simulink model "LQR_control_Xmotion"  (R2025b)
settings: Solver=VariableStepAuto  StartTime=0.0  StopTime=10.0  RelTol=1e-3
values from neighbouring files (symbols this model uses):
  A_Mat = [ 0     1    0     0   0   0 ... (first row only)    [LQR_code_XYmotion.m]    (also in LQR_code_Xmotion.m = [ 0     1    0     0; LQR_control_AND_Plant2026.m = [ 0     1    0     0)
  B_Mat = [ 0    0 ... (first row only)    [LQR_code_XYmotion.m]    (also in LQR_code_Xmotion.m = [ 0; LQR_control_AND_Plant2026.m = [ 0)
  C_Mat = [ 1  0    0   0   0  0 ... (first row only)    [LQR_code_XYmotion.m]    (also in LQR_code_Xmotion.m = [ 1  0    0   0; LQR_control_AND_Plant2026.m = [ 1  0    0   0)
  K = lqr(A_Mat, B_Mat, Q, R)    [LQR_code_XYmotion.m]    (also in LQR_code_Xmotion.m; LQR_control_AND_Plant2026.m)
settings Model: Creator=Mahmoud Essam  LastModifiedBy=Mahmoud Essam

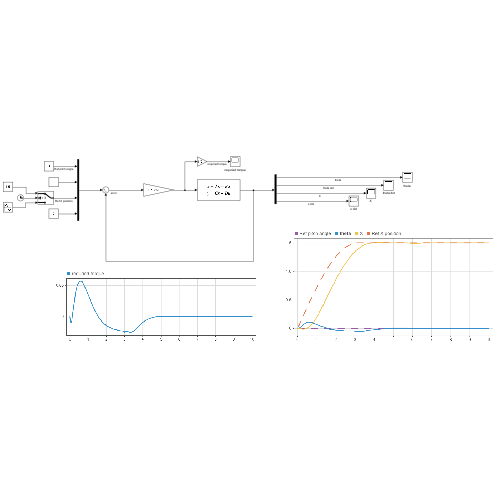
[thumbnail: Simulink's stored preview of the top-level diagram]
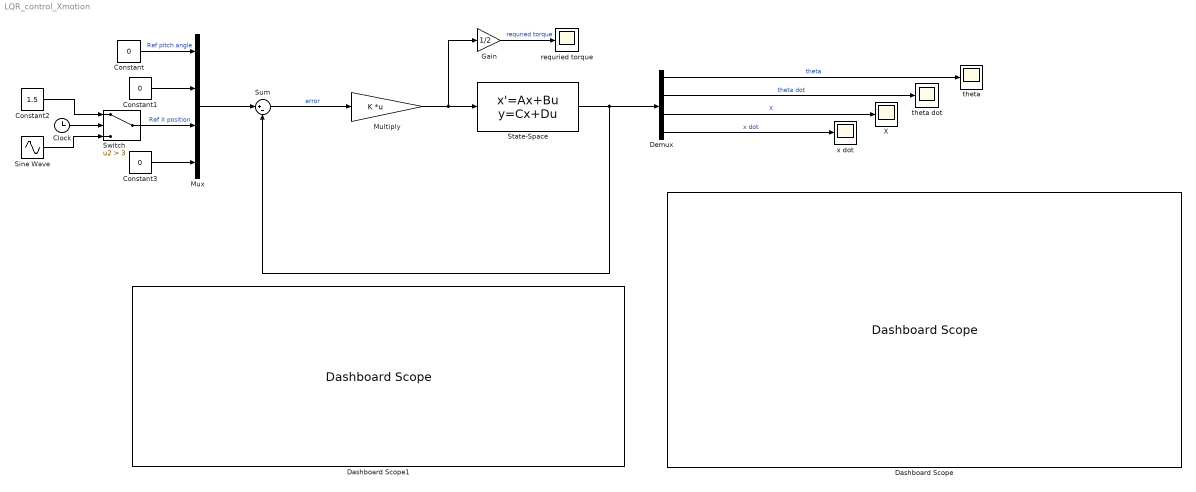
== system LQR_control_Xmotion ==
  " theta dot" : Scope
      settings: ActiveDisplayYMinimum=-22.999413149940512  ActiveDisplayYMaximum=55.548140907039681
  Clock : Clock
  Constant : Constant  Value=0
  Constant1 : Constant  Value=0
  Constant2 : Constant  Value=1.5
  Constant3 : Constant  Value=0
  Dashboard Scope : DashboardScope  FontColor=[0.0, 0.0, 0.0]
  Dashboard Scope1 : DashboardScope  FontColor=[0.0, 0.0, 0.0]
  Demux : Demux
  Gain : Gain  Gain=1/2
  Multiply : Gain  Gain=K  Multiplication=Matrix(K*u) (u vector)
  Mux : Mux
  Sine Wave : Sin  Amplitude=1.5  Frequency=.5  SampleTime=0
  State-Space : StateSpace  A=A_Mat  B=B_Mat  C=C_Mat  D=[0 ; 0 ; 0; 0]  InitialCondition=0
  Sum : Sum  Inputs=|+-
  Switch : Switch  Criteria=u2 > Threshold  Threshold=3  SaturateOnIntegerOverflow=off  InputSameDT=off
  "X " : Scope
      settings: ActiveDisplayYMinimum=-1  ActiveDisplayYMaximum=1  DataLoggingVariableName=ScopeData2
  requried torque : Scope
      settings: ActiveDisplayYMinimum=-32.84602870974846  ActiveDisplayYMaximum=12.771545913123331  DataLoggingVariableName=ScopeData4
  "theta " : Scope
      settings: ActiveDisplayYMinimum=-1  ActiveDisplayYMaximum=1
  x dot : Scope
      settings: ActiveDisplayYMinimum=-1  ActiveDisplayYMaximum=1  DataLoggingVariableName=ScopeData3
  wires:
  Demux/1 -> "theta "/1  "theta"
  Demux/2 -> " theta dot"/1  "theta dot"
  Multiply/1 -> Gain/1, State-Space/1
  Demux/4 -> x dot/1  "x dot"
  Sum/1 -> Multiply/1  "error"
  State-Space/1 -> Sum/2, Demux/1
  Demux/3 -> "X "/1  "X"
  Mux/1 -> Sum/1
  Constant3/1 -> Mux/4
  Switch/1 -> Mux/3  "Ref X position"
  Constant1/1 -> Mux/2
  Constant/1 -> Mux/1  "Ref pitch angle"
  Gain/1 -> requried torque/1  "requried torque"
  Clock/1 -> Switch/2
  Sine Wave/1 -> Switch/3
  Constant2/1 -> Switch/1
